simulink model "SCR_SiLS_R4_D101"  (R2023a)
settings: Solver=VariableStepAuto  StartTime=0.0  StopTime=T_sim_end  RelTol=1e-3
model workspace (MAT data in the model file):
  ConnVar.ipAddress = '192.168.0.153'
  ConnVar.user = 'M1'
  ConnVar.pwd = [145 145 158 146 151 156 158 157]
  ConnVar.targetHandle = 0
libraries: M1SWBlocks x6, simulink x6
settings Model: Creator=CHSE  LastModifiedBy=gione
settings DebuggingCC: UnconnectedInputMsg=warning  UnconnectedOutputMsg=warning  UnconnectedLineMsg=warning
settings ModelReferenceCC: EnableRefExpFcnMdlSchedulingChecks=on
settings RTWCC: DLArmComputeVersion=19.05

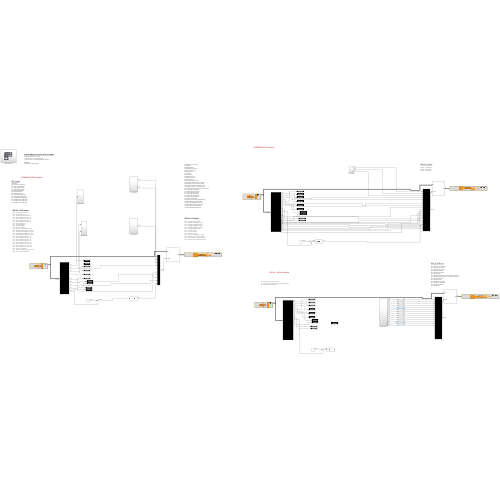
[thumbnail: Simulink's stored preview of the top-level diagram]
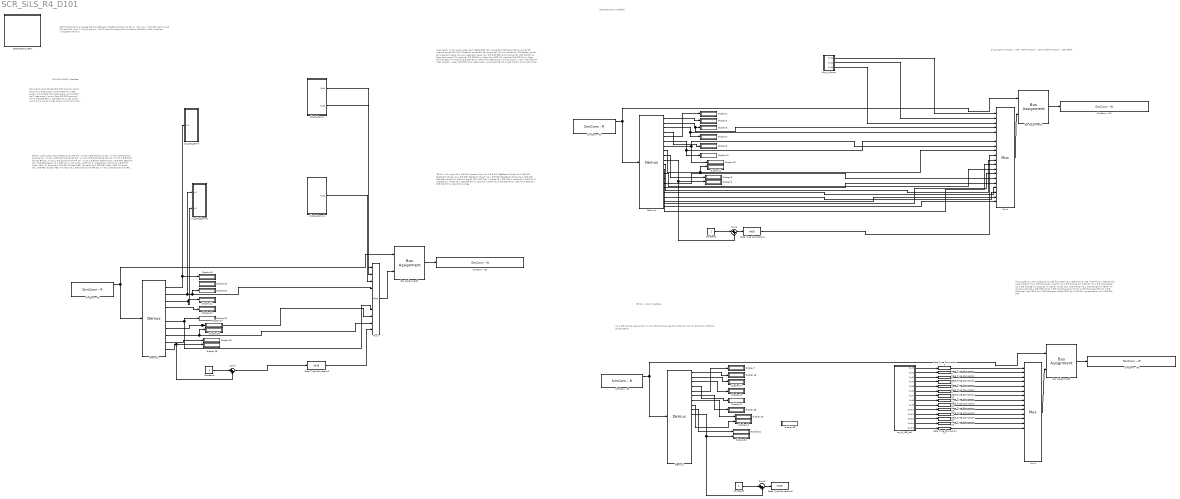
== system SCR_SiLS_R4_D101 ==
  note: No.1 G/E Dosing urea control VV
      |
      | No.1 G/E Dosing urea flow rate (l/h) (KR, NK class)
      |
      | No.1 G/E NOx concentration
  note: GE No. 1 DI intput
      |
      | No.1 G/E NOx sensor Alarm
      |
      | No.1 G/E RSV Feedback (Open)
      |
      | No.1 G/E RSV Feedback (Close)
      |
      | No.1 G/E RBV Feedback (Open)
      |
      | No.1 G/E RBV Feedback (Close)
      |
      | No.1 G/E SCR Remote mode
      |
      | No.1 G/E Run signal
      |
      | No.1 G/E Tier III mode
      |
      | No.1 G/E Tier II mode
      |
      | No.1 G/E Tier III preparation mode
      |
      | No.1 G/E SCR Em'cy stop from panel
      |
      | No.1 G/E SCR Emc'y stop from ECR
      |
      | No.1 G/E SCR Em'cy stop from bridge
  note: GE No. 1 DO output
      |
      | No.1 G/E Dosing urea Sol. VV
      |
      | No.1 G/E Dosing air Sol. VV
      |
      | No.1 G/E Dosing purging Sol. VV
      |
      | No.1 G/E Soot blower #1 Sol. VV
      |
      | No.1 G/E Soot blower #2 Sol. VV
      |
      | No.1 G/E Soot blower #3 Sol. VV
      |
      | No.1 G/E Soot blower #4 Sol. VV
      |
      | No.1 G/E RSV Setpoint
      |
      | No.1 G/E RBV Setpoint
      |
      | No.1 G/E SCR Ready
      |
      | No.1 G/E Tier III Active
      |
      | No.1 G/E Tier III preparation Active
      |
      | No.1 G/E RSV Open (ABS, NK class)
      |
      | No.1 G/E RSV Closed (ABS, NK class)
      |
      | No.1 G/E RBV Open (ABS, NK class)
      |
      | No.1 G/E RBV Closed (ABS, NK class)
      |
      | No.1 G/E Soot blower #5 Sol. VV
      |
      | No.1 G/E Soot blower #6 Sol. VV
      |
      | No.1 G/E Soot blower #7 Sol. VV
      |
      | No.1 G/E Soot blower #8 Sol. VV
      |
      | No.1 G/E Soot blower #9 Sol. VV
      |
      | No.1 G/E Soot blower #10 Sol. VV
      |
      | No.1 G/E Soot blower #11 Sol. VV
      |
      | No.1 G/E Soot blower #12 Sol. VV
      |
      | No.1 G/E Tier III Transfer
      |
      | No.1 SCR both bypass valve not open
      |
      | No.# G/E Common Shutdown
  note: DO output
      | Alarm Buzzer
      |
      | G/E SCR common alarm lamp
      |
      | No.1 Urea supply pump Start
      |
      | No.1 Urea supply pump Stop
      |
      | No.2 Urea supply pump Start
      |
      | No.2 Urea supply pump Stop
      |
      | G/E SCR common Alarm
      |
      | G/E SCR Em'cy Stopped
      |
      | No.1 Urea supply pump Running
      |
      | No.2 Urea supply pump Running
      |
      | No.1 G/E SCR Common Alarm lamp
      |
      | No.2 G/E SCR Common Alarm lamp
      |
      | No.3 G/E SCR Common Alarm lamp
      |
      | No.4 G/E SCR Common Alarm lamp
      |
      | ​
      |
      | ​
  note: Urea supply pump Auto mode
      |
      | Alarm Reset
      |
      | SCR Main power fail
      |
      | SCR Redundancy power fail
      |
      | Internal power fail(삭제됨)
      |
      | External power fail
      |
      | Fan power fail
      |
      | DC low insulation
      |
      | UPS battery power fail
      |
      | Urea tank Level Low-Low
      |
      | Urea tank Level Low
      |
      | G/E SCR ESD circuit power fail
      |
      | G/E SCR Em'cy Stop From panel (To module)
      |
      | G/E SCR Em'cy Stop From ECR (To module)
      |
      | G/E SCR Em'cy Stop From Bridge (To module)
      |
      | G/E SCR Em'cy Stop From Near Supply pump
      |
      | Supply, urea inlet filter dP High (Supply, urea inlet PDS)
      |
      | No.1 Urea supply pump Remote
      |
      | No.1 Urea supply pump Abnormal
      |
      | No.1 Urea supply pump Running
      |
      | No.2 Urea supply pump Remote
      |
      | No.2 Urea supply pump Abnormal
      |
      | No.2 Urea supply pump Running
      |
      | G/E Low Sulfur fuel supplied
      |
      | Urea tank drip tray Level High-High (ABS class)
      |
      | Urea tank TEMP High-High (ABS class)
      |
      | Urea tank Level High (ABS, BV, NK class)
      |
      | Urea tank drip tray Level High (ABS class)
      |
      | Urea tank TEMP Low (ABS, NK class)
      |
      | Urea tank TEMP High (ABS, NK class)
      |
      | ​
      |
      | ​
  note: COMMON DO/DI Interface
  note: SCR SiLS Model to evaluate the PLC software
      | modified at 2024.04.18. by Y.B. Kim
      |
      | -> Sils_DO_Comm: PLC DO and Sils input
      | -> Sils_DI_Comm : PLC DI and Sils output for simulation
      |
      | REMARK!!!
      | first, initialize workspace memory
  note: COMMON AO/AI Interface
  note: Sils_AI_Comm
      |
      | Supply, urea inlet PT
      |
      | Supply, urea outlet PT
      |
      | Supply, urea TEMP
  note: Sils_AI_GE no 1
      |
      | No.1 G/E Dosing urea flowmeter
      |
      | No.1 G/E Dosing urea inlet PT
      |
      | No.1 G/E Dosing urea outlet PT
      |
      | No.1 G/E Dosing air inlet PT
      |
      | No.1 G/E Dosing air outlet PT
      |
      | No.1 G/E Load signal
      |
      | No.1 G/E Charge Air pressure, Air cooler outlet (No.1 G/E PT212)
      |
      | No.1 G/E Charge Air TEMP, Air cooler outlet (No.1 G/E TE212)
      |
      | No.1 G/E Soot blower air PT
      |
      | No.1 G/E Chamber PDT
      |
      | No.1 G/E Chamber inlet TEMP
      |
      | No.1 G/E Chamber outlet TEMP
      |
      | No.1 G/E NOx concentration
      |
      | No.1 G/E RBV PDT
      |
      | ​
      |
      | ​
  note: GE No. 1 AO/AI Interface
  Bus Assignment1 : BusAssignment  AssignedSignals=data
  Bus Assignment2 : BusAssignment  AssignedSignals=data
  Bus Assignment3 : BusAssignment  AssignedSignals=data
  Constant1 : Constant
  Constant2 : Constant
  Constant3 : Constant
  Dashboard-system : Subsystem
  Data Type Conversion{1..17} (17 alike) : DataTypeConversion  OutDataTypeStr=int16  SaturateOnIntegerOverflow=off  RndMeth=Floor
  Demux1 : Demux  Outputs=20
  Demux2 : Demux  Outputs=10
  Demux4 : Demux  Outputs=20
  Display{1..5,7..32} (31 alike) : Display
      Display17 settings: Format=decimal (Stored Integer)
      Display20 settings: Format=decimal (Stored Integer)
      Display3 settings: Format=decimal (Stored Integer)
  Mux1 : Mux  Inputs=20
  Mux2 : Mux  Inputs=10
  Mux4 : Mux  Inputs=20
  SimConn - R1 : M1SWBlocks/SimConn Blocks/SimConn - R  connVarName=ConnVar  InswModuleName='NONOXR4'  swModuleName=NONOXR4  InvarName='.Sils_AO_Comm'  varName=.Sils_AO_Comm  varDataType=Bus: IOSim_AIO_typ  enRetOutput=on  enGetTrigger=off  getTrigger=rising  valDurLostConn=Zero  internalVal=0  DataDim=1  enSampTimMon=on  sampleTime=Ts_com
      settings: SourceProductName=Bachmann M1 Software
  SimConn - R2 : M1SWBlocks/SimConn Blocks/SimConn - R  connVarName=ConnVar  InswModuleName='NONOXR4'  swModuleName=NONOXR4  InvarName='.Sils_DO_Comm'  varName=.Sils_DO_Comm  varDataType=Bus: IOSim_typ  enRetOutput=on  enGetTrigger=off  getTrigger=rising  valDurLostConn=Zero  internalVal=0  DataDim=1  enSampTimMon=on  sampleTime=Ts_com
      settings: SourceProductName=Bachmann M1 Software
  SimConn - R3 : M1SWBlocks/SimConn Blocks/SimConn - R  connVarName=ConnVar  InswModuleName='NONOXR4'  swModuleName=NONOXR4  InvarName='.Sils_AO_GE1'  varName=.Sils_AO_GE1  varDataType=Bus: IOSim_AIO_typ  enRetOutput=on  enGetTrigger=off  getTrigger=rising  valDurLostConn=Zero  internalVal=0  DataDim=1  enSampTimMon=on  sampleTime=Ts_com
      settings: SourceProductName=Bachmann M1 Software
  SimConn - W1 : M1SWBlocks/SimConn Blocks/SimConn - W  connVarName=ConnVar  InswModuleName='NONOXR4'  swModuleName=NONOXR4  InvarName='.Sils_AI_Comm'  varName=.Sils_AI_Comm  varDataType=Bus: IOSim_AIO_typ  enRetOutput=off  enGetTrigger=off  getTrigger=rising  enSampTimMon=off
      settings: SourceProductName=Bachmann M1 Software
  SimConn - W2 : M1SWBlocks/SimConn Blocks/SimConn - W  connVarName=ConnVar  InswModuleName='NONOXR4'  swModuleName=NONOXR4  InvarName='.Sils_DI_Comm'  varName=.Sils_DI_Comm  varDataType=Bus: IOSim_typ  enRetOutput=off  enGetTrigger=off  getTrigger=rising  enSampTimMon=off
      settings: SourceProductName=Bachmann M1 Software
  SimConn - W3 : M1SWBlocks/SimConn Blocks/SimConn - W  connVarName=ConnVar  InswModuleName='NONOXR4'  swModuleName=NONOXR4  InvarName='.Sils_AI_GE1'  varName=.Sils_AI_GE1  varDataType=Bus: IOSim_AIO_typ  enRetOutput=off  enGetTrigger=off  getTrigger=rising  enSampTimMon=off
      settings: SourceProductName=Bachmann M1 Software
  Sum1 : Sum  Inputs=|++
  Sum2 : Sum  Inputs=|++
  Sum3 : Sum  Inputs=|++
  sils_AI_Comm : Subsystem
  sils_AI_GE_No1 : Subsystem
  sils_DI_Comm : Subsystem
  sils_DI_Comm1 : Subsystem
  sils_DO_Comm : Subsystem
  sils_DO_Comm1 : Subsystem
  wires:
  Demux2/3 -> sils_DO_Comm1/2(In2), Display21/1
  Constant1/1 -> Sum1/1
  Demux2/4 -> Display22/1
  Sum1/1 -> Data Type Conversion2/1
  Demux2/2 -> Mux2/4, Display20/1, sils_DO_Comm1/1(In1)
  SimConn - R2/1 -> Bus Assignment2/1, Demux2/1
  Demux2/9 -> Display25/1
  Demux2/10 -> Sum1/2, Display26/1
  Demux2/8 -> Mux2/9, Display28/1
  Demux2/7 -> Mux2/8, Display27/1
  Demux2/6 -> Mux2/7, Display29/1
  Mux2/1 -> Bus Assignment2/2
  Bus Assignment2/1 -> SimConn - W2/1
  Data Type Conversion2/1 -> Mux2/10
  Demux4/6 -> Display12/1, Mux4/7
  Bus Assignment1/1 -> SimConn - W1/1
  Demux4/9 -> Display8/1
  Demux4/7 -> Display10/1, Mux4/8
  Mux4/1 -> Bus Assignment1/2
  Demux4/10 -> Sum2/2, Display9/1
  Demux4/1 -> Display2/1
  Data Type Conversion1/1 -> Mux4/10
  Demux4/8 -> Mux4/9, Display11/1
  Demux4/5 -> Display1/1
  SimConn - R1/1 -> Bus Assignment1/1, Demux4/1
  Demux4/4 -> Display5/1
  Demux4/2 -> Mux4/4, Display3/1
  Sum2/1 -> Data Type Conversion1/1
  Constant2/1 -> Sum2/1
  Demux4/3 -> Display4/1, Mux4/5
  Demux4/11 -> Mux4/11
  Demux4/12 -> Mux4/12
  Demux4/13 -> Mux4/13
  Demux4/14 -> Mux4/14
  Demux4/15 -> Mux4/15
  Demux4/16 -> Mux4/16
  Demux4/17 -> Mux4/17
  Demux4/18 -> Mux4/18
  Demux4/19 -> Mux4/19
  Demux4/20 -> Mux4/20
  Demux2/1 -> sils_DO_Comm/1(In1), Display18/1
  sils_DI_Comm/1(Out2) -> Mux2/1
  sils_DI_Comm/2(Out3) -> Mux2/2
  sils_AI_Comm/1(Out1) -> Mux4/1
  sils_AI_Comm/2(Out2) -> Mux4/2
  sils_AI_Comm/3(Out3) -> Mux4/3
  sils_DI_Comm1/1(Out2) -> Mux2/3
  Constant3/1 -> Sum3/1
  Demux1/1 -> Display16/1
  Demux1/4 -> Display24/1
  Demux1/5 -> Display7/1
  Demux1/2 -> Display17/1
  Demux1/9 -> Display31/1
  Mux1/1 -> Bus Assignment3/2
  Bus Assignment3/1 -> SimConn - W3/1
  Demux1/6 -> Display15/1
  Sum3/1 -> Data Type Conversion3/1
  Demux1/8 -> Display14/1
  Demux1/7 -> Display13/1
  SimConn - R3/1 -> Bus Assignment3/1, Demux1/1
  Demux1/3 -> Display23/1
  sils_AI_GE_No1/3(Out3) -> Data Type Conversion6/1
  sils_AI_GE_No1/1(Out1) -> Data Type Conversion4/1
  sils_AI_GE_No1/2(Out2) -> Data Type Conversion5/1
  Demux1/10 -> Sum3/2, Display32/1
  sils_AI_GE_No1/4(Out4) -> Data Type Conversion7/1
  sils_AI_GE_No1/5(Out5) -> Data Type Conversion8/1
  sils_AI_GE_No1/6(Out6) -> Data Type Conversion9/1
  sils_AI_GE_No1/7(Out7) -> Data Type Conversion10/1
  sils_AI_GE_No1/8(Out8) -> Data Type Conversion11/1
  sils_AI_GE_No1/9(Out9) -> Data Type Conversion12/1
  sils_AI_GE_No1/10(Out10) -> Data Type Conversion13/1
  sils_AI_GE_No1/11(Out11) -> Data Type Conversion14/1
  sils_AI_GE_No1/12(Out12) -> Data Type Conversion15/1
  sils_AI_GE_No1/14(Out13) -> Data Type Conversion17/1
  sils_AI_GE_No1/13(Out14) -> Data Type Conversion16/1
  Data Type Conversion4/1 -> Mux1/1
  Data Type Conversion5/1 -> Mux1/2
  Data Type Conversion6/1 -> Mux1/3
  Data Type Conversion9/1 -> Mux1/6
  Data Type Conversion8/1 -> Mux1/5
  Data Type Conversion7/1 -> Mux1/4
  Data Type Conversion10/1 -> Mux1/7
  Data Type Conversion11/1 -> Mux1/8
  Data Type Conversion12/1 -> Mux1/9
  Data Type Conversion13/1 -> Mux1/10
  Data Type Conversion14/1 -> Mux1/11
  Data Type Conversion15/1 -> Mux1/12
  Data Type Conversion16/1 -> Mux1/13
  Data Type Conversion17/1 -> Mux1/14

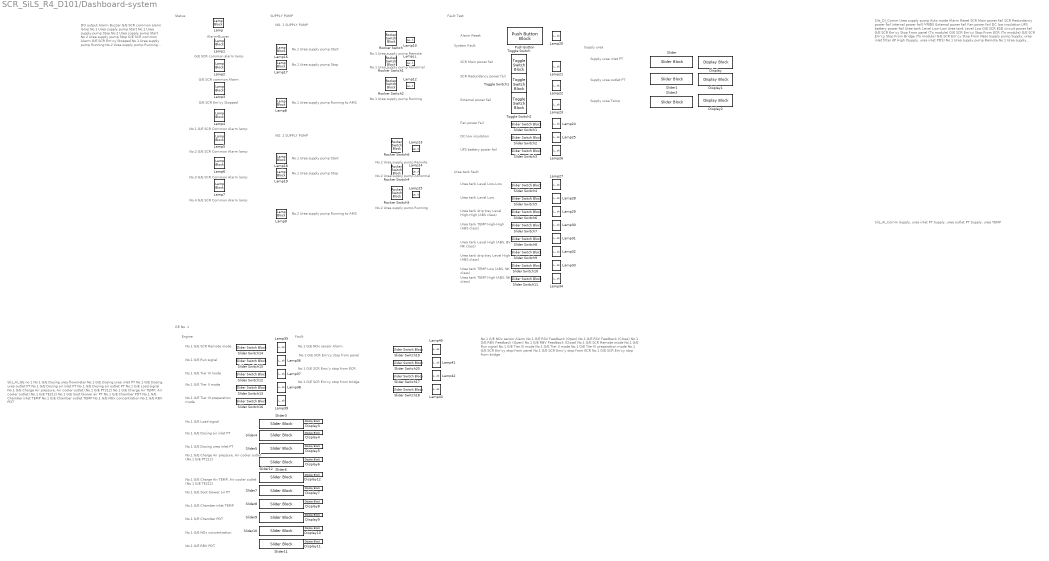
== system SCR_SiLS_R4_D101/Dashboard-system ==
  note: Fault
  note: Engine
  note: GE No. 1
  note: Supply urea
  note: Urea tank fault
  note: System Fault
  note: NO. 1 SUPPLY PUMP
  note: SUPPLY PUMP
  note: Alarm Buzzer
  note: G/E SCR common alarm lamp
  note: DO output
      | Alarm Buzzer
      |
      | G/E SCR common alarm lamp
      |
      | No.1 Urea supply pump Start
      |
      | No.1 Urea supply pump Stop
      |
      | No.2 Urea supply pump Start
      |
      | No.2 Urea supply pump Stop
      |
      | G/E SCR common Alarm
      |
      | G/E SCR Em'cy Stopped
      |
      | No.1 Urea supply pump Running
      |
      | No.2 Urea supply pump Running
      |
      | No.1 G/E SCR Common Alarm lamp
      |
      | No.2 G/E SCR Common Alarm lamp
      |
      | No.3 G/E SCR Common Alarm lamp
      |
      | No.4 G/E SCR Common Alarm lamp
      |
      | ​
      |
      | ​
  note: G/E SCR Em'cy Stopped
  note: G/E SCR common Alarm
  note: No.1 G/E SCR Common Alarm lamp
  note: No.2 G/E SCR Common Alarm lamp
  note: No.3 G/E SCR Common Alarm lamp
  note: No.4 G/E SCR Common Alarm lamp
  note: Status
  note: No.1 Urea supply pump Running to AMS
  note: NO. 2 SUPPLY PUMP
  note: No.2 Urea supply pump Running to AMS
  note: No.1 Urea supply pump Remote
  note: No.1 Urea supply pump Abnormal
  note: No.1 Urea supply pump Running
  note: Sils_DI_Comm
      |
      | Urea supply pump Auto mode
      |
      | Alarm Reset
      |
      | SCR Main power fail
      |
      | SCR Redundancy power fail
      |
      | Internal power fail(삭제됨)
      |
      | External power fail
      |
      | Fan power fail
      |
      | DC low insulation
      |
      | UPS battery power fail
      |
      | Urea tank Level Low-Low
      |
      | Urea tank Level Low
      |
      | G/E SCR ESD circuit power fail
      |
      | G/E SCR Em'cy Stop From panel (To module)
      |
      | G/E SCR Em'cy Stop From ECR (To module)
      |
      | G/E SCR Em'cy Stop From Bridge (To module)
      |
      | G/E SCR Em'cy Stop From Near Supply pump
      |
      | Supply, urea inlet filter dP High (Supply, urea inlet PDS)
      |
      | No.1 Urea supply pump Remote
      |
      | No.1 Urea supply pump Abnormal
      |
      | No.1 Urea supply pump Running
      |
      | No.2 Urea supply pump Remote
      |
      | No.2 Urea supply pump Abnormal
      |
      | No.2 Urea supply pump Running
      |
      | G/E Low Sulfur fuel supplied
      |
      | Urea tank drip tray Level High-High (ABS class)
      |
      | Urea tank TEMP High-High (ABS class)
      |
      | Urea tank Level High (ABS, BV, NK class)
      |
      | Urea tank drip tray Level High (ABS class)
      |
      | Urea tank TEMP Low (ABS, NK class)
      |
      | Urea tank TEMP High (ABS, NK class)
      |
      | ​
      |
      | ​
  note: No.2 Urea supply pump Running
  note: No.2 Urea supply pump Abnormal
  note: No.2 Urea supply pump Remote
  note: No.1 Urea supply pump Start
  note: No.1 Urea supply pump Stop
  note: No.1 Urea supply pump Stop
  note: No.1 Urea supply pump Start
  note: Fault Test
  note: Alarm Reset
  note: SCR Main power fail
  note: SCR Redundancy power fail
  note: External power fail
  note: Fan power fail
  note: DC low insulation
  note: UPS battery power fail
  note: Urea tank Level Low-Low
  note: Urea tank Level Low
  note: Urea tank drip tray Level High-High (ABS class)
  note: Urea tank TEMP High-High (ABS class)
  note: Urea tank Level High (ABS, BV, NK class)
  note: Urea tank drip tray Level High (ABS class)
  note: Urea tank TEMP Low (ABS, NK class)
  note: Urea tank TEMP High (ABS, NK class)
  note: Supply urea inlet PT
  note: Sils_AI_Comm
      |
      | Supply, urea inlet PT
      |
      | Supply, urea outlet PT
      |
      | Supply, urea TEMP
  note: Supply urea outlet PT
  note: Supply urea Temp
  note: No.1 G/E NOx sensor Alarm
      |
      | No.1 G/E RSV Feedback (Open)
      |
      | No.1 G/E RSV Feedback (Close)
      |
      | No.1 G/E RBV Feedback (Open)
      |
      | No.1 G/E RBV Feedback (Close)
      |
      | No.1 G/E SCR Remote mode
      |
      | No.1 G/E Run signal
      |
      | No.1 G/E Tier III mode
      |
      | No.1 G/E Tier II mode
      |
      | No.1 G/E Tier III preparation mode
      |
      | No.1 G/E SCR Em'cy stop from panel
      |
      | No.1 G/E SCR Emc'y stop from ECR
      |
      | No.1 G/E SCR Em'cy stop from bridge
  note: No.1 G/E Tier II mode
  note: No.1 G/E Tier III mode
  note: No.1 G/E Run signal
  note: No.1 G/E SCR Remote mode
  note: No.1 G/E Tier III preparation mode
  note: No.1 G/E SCR Emc'y stop from ECR
  note: No.1 G/E SCR Em'cy stop from bridge
  note: No.1 G/E NOx sensor Alarm
  note: No.1 G/E SCR Em'cy stop from panel
  note: No.1 G/E Load signal
  note: Sils_AI_GE no 1
      |
      | No.1 G/E Dosing urea flowmeter
      |
      | No.1 G/E Dosing urea inlet PT
      |
      | No.1 G/E Dosing urea outlet PT
      |
      | No.1 G/E Dosing air inlet PT
      |
      | No.1 G/E Dosing air outlet PT
      |
      | No.1 G/E Load signal
      |
      | No.1 G/E Charge Air pressure, Air cooler outlet (No.1 G/E PT212)
      |
      | No.1 G/E Charge Air TEMP, Air cooler outlet (No.1 G/E TE212)
      |
      | No.1 G/E Soot blower air PT
      |
      | No.1 G/E Chamber PDT
      |
      | No.1 G/E Chamber inlet TEMP
      |
      | No.1 G/E Chamber outlet TEMP
      |
      | No.1 G/E NOx concentration
      |
      | No.1 G/E RBV PDT
      |
      | ​
      |
      | ​
  note: No.1 G/E Dosing air inlet PT
  note: No.1 G/E Dosing urea inlet PT
  note: No.1 G/E Charge Air pressure, Air cooler outlet (No.1 G/E PT212)
  note: No.1 G/E Soot blower air PT
  note: No.1 G/E Chamber inlet TEMP
  note: No.1 G/E Chamber PDT
  note: No.1 G/E NOx concentration
  note: No.1 G/E RBV PDT
  note: No.1 G/E Charge Air TEMP, Air cooler outlet (No.1 G/E TE212)
  Display{,1..12} (13 alike) : DisplayBlock  LabelPosition=Hide  Transparency=1
  Lamp{,1..43} (44 alike) : LampBlock  LabelPosition=Hide
  Push Button : PushButtonBlock  ButtonText=Alarm Reset  OffValue=0.000000
  Rocker Switch{,1..2,4..6} (6 alike) : RockerSwitchBlock  LabelPosition=Hide
      settings: Values={{'Off', 'On'}, [0 1]}
  Slider : SliderBlock  LabelPosition=Hide  ScaleMax=16
  Slider Switch{1..20} (20 alike) : SliderSwitchBlock  LabelPosition=Hide
      settings: Values={{'Off', 'On'}, [0 1]}
  Slider1 : SliderBlock  LabelPosition=Hide  ScaleMax=16
  Slider10 : SliderBlock  LabelPosition=Hide  ScaleMax=120
  Slider11 : SliderBlock  LabelPosition=Hide
  Slider12 : SliderBlock  LabelPosition=Hide  ScaleMax=200
  Slider2 : SliderBlock  LabelPosition=Hide
  Slider3 : SliderBlock  LabelPosition=Hide  ScaleMax=120
  Slider4 : SliderBlock  LabelPosition=Hide  ScaleMax=15
  Slider5 : SliderBlock  LabelPosition=Hide  ScaleMax=15
  Slider6 : SliderBlock  LabelPosition=Hide  ScaleMax=10
  Slider7 : SliderBlock  LabelPosition=Hide  ScaleMax=120
  Slider8 : SliderBlock  LabelPosition=Hide  ScaleMax=600
  Slider9 : SliderBlock  LabelPosition=Hide
  Toggle Switch : ToggleSwitchBlock  LabelPosition=Hide
      settings: Values={{'Off', 'On'}, [0 1]}
  Toggle Switch1 : ToggleSwitchBlock  LabelPosition=Hide
      settings: Values={{'Off', 'On'}, [0 1]}
  Toggle Switch2 : ToggleSwitchBlock  LabelPosition=Hide
      settings: Values={{'Off', 'On'}, [0 1]}

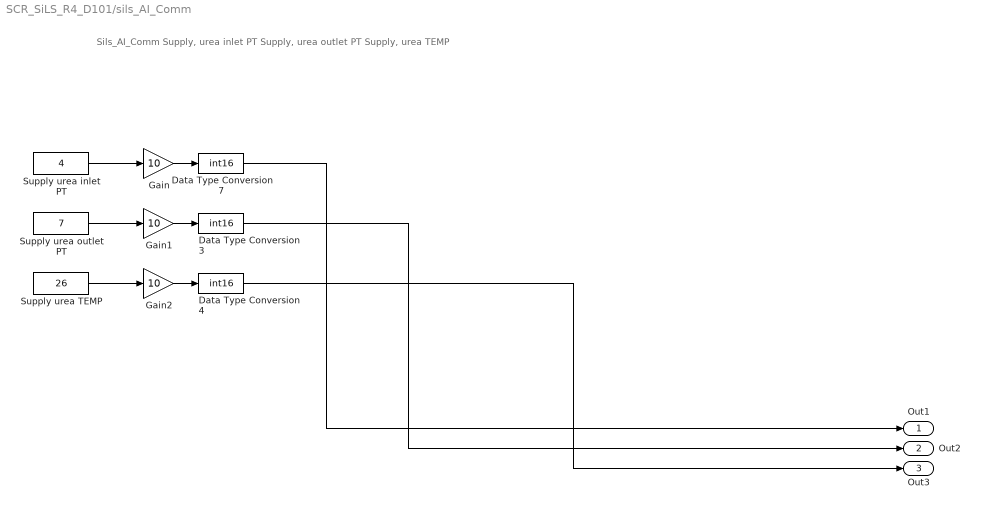
== system SCR_SiLS_R4_D101/sils_AI_Comm ==
  note: Sils_AI_Comm
      |
      | Supply, urea inlet PT
      |
      | Supply, urea outlet PT
      |
      | Supply, urea TEMP
  Data Type Conversion3 : DataTypeConversion  OutDataTypeStr=int16  SaturateOnIntegerOverflow=off  RndMeth=Floor
  Data Type Conversion4 : DataTypeConversion  OutDataTypeStr=int16  SaturateOnIntegerOverflow=off  RndMeth=Floor
  Data Type Conversion7 : DataTypeConversion  OutDataTypeStr=int16  SaturateOnIntegerOverflow=off  RndMeth=Floor
  Gain : Gain  Gain=10
  Gain1 : Gain  Gain=10
  Gain2 : Gain  Gain=10
  Supply urea TEMP : Constant  Value=26
  Supply urea inlet PT : Constant  Value=4
  Supply urea outlet PT : Constant  Value=7
  Out1 : Outport
  Out2 : Outport  Port=2
  Out3 : Outport  Port=3
  wires:
  Supply urea inlet PT/1 -> Gain/1
  Supply urea outlet PT/1 -> Gain1/1
  Gain1/1 -> Data Type Conversion3/1
  Data Type Conversion3/1 -> Out2/1
  Supply urea TEMP/1 -> Gain2/1
  Gain2/1 -> Data Type Conversion4/1
  Gain/1 -> Data Type Conversion7/1
  Data Type Conversion7/1 -> Out1/1
  Data Type Conversion4/1 -> Out3/1

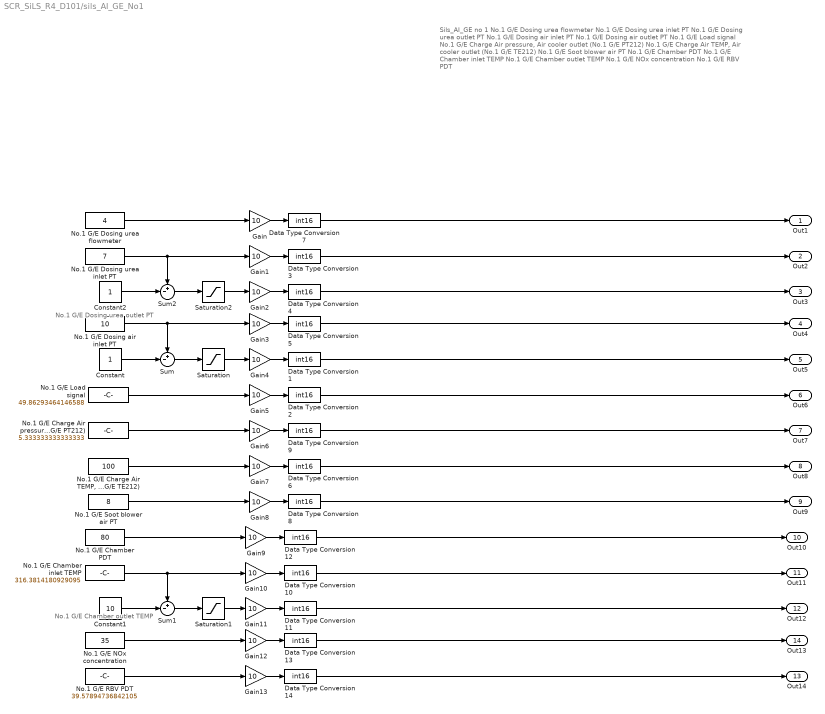
== system SCR_SiLS_R4_D101/sils_AI_GE_No1 ==
  note: No.1 G/E Dosing urea outlet PT
  note: No.1 G/E Chamber outlet TEMP
  note: Sils_AI_GE no 1
      |
      | No.1 G/E Dosing urea flowmeter
      |
      | No.1 G/E Dosing urea inlet PT
      |
      | No.1 G/E Dosing urea outlet PT
      |
      | No.1 G/E Dosing air inlet PT
      |
      | No.1 G/E Dosing air outlet PT
      |
      | No.1 G/E Load signal
      |
      | No.1 G/E Charge Air pressure, Air cooler outlet (No.1 G/E PT212)
      |
      | No.1 G/E Charge Air TEMP, Air cooler outlet (No.1 G/E TE212)
      |
      | No.1 G/E Soot blower air PT
      |
      | No.1 G/E Chamber PDT
      |
      | No.1 G/E Chamber inlet TEMP
      |
      | No.1 G/E Chamber outlet TEMP
      |
      | No.1 G/E NOx concentration
      |
      | No.1 G/E RBV PDT
      |
      | ​
      |
      | ​
  Constant : Constant
  Constant1 : Constant  Value=10
  Constant2 : Constant
  Data Type Conversion{1..14} (14 alike) : DataTypeConversion  OutDataTypeStr=int16  SaturateOnIntegerOverflow=off  RndMeth=Floor
  Gain{,1..13} (14 alike) : Gain  Gain=10
  No.1 G/E Chamber PDT : Constant  Value=80
  No.1 G/E Chamber inlet TEMP : Constant  Value=316.3814180929095
  "No.1 G/E Charge Air TEMP, Air cooler outlet (No.1 G/E TE212)" : Constant  Value=100
  "No.1 G/E Charge Air pressure, Air cooler outlet (No.1 G/E PT212)" : Constant  Value=5.333333333333333
  No.1 G/E Dosing air inlet PT : Constant  Value=10
  No.1 G/E Dosing urea flowmeter : Constant  Value=4
  No.1 G/E Dosing urea inlet PT : Constant  Value=7
  No.1 G/E Load signal : Constant  Value=49.86293464146588
  No.1 G/E NOx concentration : Constant  Value=35
  No.1 G/E RBV PDT : Constant  Value=39.57894736842105
  No.1 G/E Soot blower air PT : Constant  Value=8
  Saturation : Saturate  UpperLimit=10.0  LowerLimit=0.0
  Saturation1 : Saturate  UpperLimit=500.0  LowerLimit=0.0
  Saturation2 : Saturate  UpperLimit=10.0  LowerLimit=0.0
  Sum : Sum  Inputs=+-|
  Sum1 : Sum  Inputs=+-|
  Sum2 : Sum  Inputs=+-|
  Out1 : Outport
  Out2 : Outport  Port=2
  Out3 : Outport  Port=3
  Out4 : Outport  Port=4
  Out5 : Outport  Port=5
  Out6 : Outport  Port=6
  Out7 : Outport  Port=7
  Out8 : Outport  Port=8
  Out9 : Outport  Port=9
  Out10 : Outport  Port=10
  Out11 : Outport  Port=11
  Out12 : Outport  Port=12
  Out14 : Outport  Port=13
  Out13 : Outport  Port=14
  wires:
  No.1 G/E Dosing urea flowmeter/1 -> Gain/1
  Gain1/1 -> Data Type Conversion3/1
  Data Type Conversion3/1 -> Out2/1
  Gain2/1 -> Data Type Conversion4/1
  Gain/1 -> Data Type Conversion7/1
  Data Type Conversion7/1 -> Out1/1
  Data Type Conversion4/1 -> Out3/1
  No.1 G/E Dosing air inlet PT/1 -> Gain3/1, Sum/1
  Gain4/1 -> Data Type Conversion1/1
  Sum/1 -> Saturation/1
  No.1 G/E Load signal/1 -> Gain5/1
  Data Type Conversion5/1 -> Out4/1
  Data Type Conversion1/1 -> Out5/1
  Data Type Conversion2/1 -> Out6/1
  Gain3/1 -> Data Type Conversion5/1
  Gain5/1 -> Data Type Conversion2/1
  "No.1 G/E Charge Air pressure, Air cooler outlet (No.1 G/E PT212)"/1 -> Gain6/1
  Gain7/1 -> Data Type Conversion6/1
  "No.1 G/E Charge Air TEMP, Air cooler outlet (No.1 G/E TE212)"/1 -> Gain7/1
  No.1 G/E Soot blower air PT/1 -> Gain8/1
  Data Type Conversion9/1 -> Out7/1
  Data Type Conversion6/1 -> Out8/1
  Data Type Conversion8/1 -> Out9/1
  Gain6/1 -> Data Type Conversion9/1
  Gain8/1 -> Data Type Conversion8/1
  No.1 G/E Chamber PDT/1 -> Gain9/1
  Gain10/1 -> Data Type Conversion10/1
  No.1 G/E Chamber inlet TEMP/1 -> Sum1/1, Gain10/1
  Data Type Conversion12/1 -> Out10/1
  Data Type Conversion10/1 -> Out11/1
  Data Type Conversion11/1 -> Out12/1
  Gain9/1 -> Data Type Conversion12/1
  Gain11/1 -> Data Type Conversion11/1
  No.1 G/E RBV PDT/1 -> Gain13/1
  Data Type Conversion14/1 -> Out14/1
  Data Type Conversion13/1 -> Out13/1
  Gain12/1 -> Data Type Conversion13/1
  Gain13/1 -> Data Type Conversion14/1
  No.1 G/E NOx concentration/1 -> Gain12/1
  Constant/1 -> Sum/2
  Saturation/1 -> Gain4/1
  Sum1/1 -> Saturation1/1
  Constant1/1 -> Sum1/2
  Saturation1/1 -> Gain11/1
  No.1 G/E Dosing urea inlet PT/1 -> Gain1/1, Sum2/1
  Sum2/1 -> Saturation2/1
  Constant2/1 -> Sum2/2
  Saturation2/1 -> Gain2/1

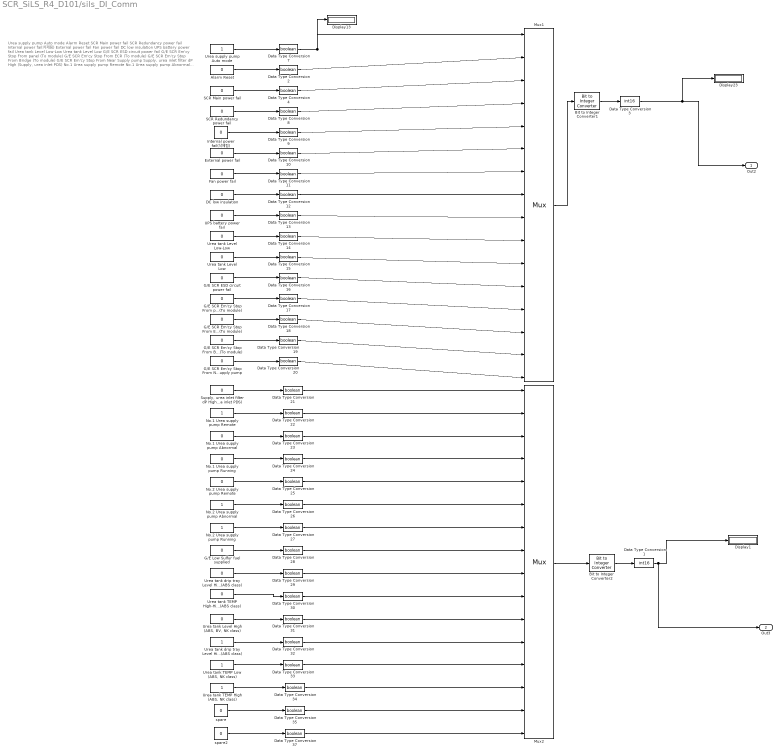
== system SCR_SiLS_R4_D101/sils_DI_Comm ==
  note: Urea supply pump Auto mode
      |
      | Alarm Reset
      |
      | SCR Main power fail
      |
      | SCR Redundancy power fail
      |
      | Internal power fail(삭제됨)
      |
      | External power fail
      |
      | Fan power fail
      |
      | DC low insulation
      |
      | UPS battery power fail
      |
      | Urea tank Level Low-Low
      |
      | Urea tank Level Low
      |
      | G/E SCR ESD circuit power fail
      |
      | G/E SCR Em'cy Stop From panel (To module)
      |
      | G/E SCR Em'cy Stop From ECR (To module)
      |
      | G/E SCR Em'cy Stop From Bridge (To module)
      |
      | G/E SCR Em'cy Stop From Near Supply pump
      |
      | Supply, urea inlet filter dP High (Supply, urea inlet PDS)
      |
      | No.1 Urea supply pump Remote
      |
      | No.1 Urea supply pump Abnormal
      |
      | No.1 Urea supply pump Running
      |
      | No.2 Urea supply pump Remote
      |
      | No.2 Urea supply pump Abnormal
      |
      | No.2 Urea supply pump Running
      |
      | G/E Low Sulfur fuel supplied
      |
      | Urea tank drip tray Level High-High (ABS class)
      |
      | Urea tank TEMP High-High (ABS class)
      |
      | Urea tank Level High (ABS, BV, NK class)
      |
      | Urea tank drip tray Level High (ABS class)
      |
      | Urea tank TEMP Low (ABS, NK class)
      |
      | Urea tank TEMP High (ABS, NK class)
      |
      | ​
      |
      | ​
  Alarm Reset : Constant  Value=0
  Bit to Integer Converter1 : simulink/Logic and Bit Operations/Bit to Integer Converter  nbits=16  bitOrder=LSB first  signedOutputValues=Unsigned  outDtype=Inherit via internal rule  outDtypeSigned=Inherit via internal rule
  Bit to Integer Converter2 : simulink/Logic and Bit Operations/Bit to Integer Converter  nbits=16  bitOrder=LSB first  signedOutputValues=Unsigned  outDtype=Inherit via internal rule  outDtypeSigned=Inherit via internal rule
  DC low insulation : Constant  Value=0
  Data Type Conversion1 : DataTypeConversion  OutDataTypeStr=int16  SaturateOnIntegerOverflow=off  RndMeth=Floor
  Data Type Conversion{2,4,7..35,37} (32 alike) : DataTypeConversion  OutDataTypeStr=boolean  SaturateOnIntegerOverflow=off  RndMeth=Floor
  Data Type Conversion3 : DataTypeConversion  OutDataTypeStr=int16  SaturateOnIntegerOverflow=off  RndMeth=Floor
  Display1 : Display
  Display13 : Display
  Display23 : Display
  External power fail : Constant  Value=0
  Fan power fail : Constant  Value=0
  G/E Low Sulfur fuel supplied : Constant  Value=0
  G/E SCR ESD circuit power fail : Constant  Value=0
  G/E SCR Em'cy Stop From Bridge (To module) : Constant  Value=0
  G/E SCR Em'cy Stop From ECR (To module) : Constant  Value=0
  G/E SCR Em'cy Stop From Near Supply pump : Constant  Value=0
  G/E SCR Em'cy Stop From panel (To module) : Constant  Value=0
  Internal power fail(삭제됨) : Constant  Value=0
  Mux1 : Mux  Inputs=16
  Mux2 : Mux  Inputs=16
  No.1 Urea supply pump Abnormal : Constant  Value=0
  No.1 Urea supply pump Remote : Constant
  No.1 Urea supply pump Running : Constant  Value=0
  No.2 Urea supply pump Abnormal : Constant
  No.2 Urea supply pump Remote : Constant  Value=0
  No.2 Urea supply pump Running : Constant
  SCR Main power fail : Constant  Value=0
  SCR Redundancy power fail : Constant  Value=0
  "Supply, urea inlet filter dP High (Supply, urea inlet PDS)" : Constant  Value=0
  UPS battery power fail : Constant  Value=0
  Urea supply pump Auto mode : Constant
  "Urea tank Level High (ABS, BV, NK class)" : Constant  Value=0
  Urea tank Level Low : Constant  Value=0
  Urea tank Level Low-Low : Constant  Value=0
  "Urea tank TEMP High (ABS, NK class)" : Constant
  Urea tank TEMP High-High (ABS class) : Constant  Value=0
  "Urea tank TEMP Low (ABS, NK class)" : Constant
  Urea tank drip tray Level High (ABS class) : Constant
  Urea tank drip tray Level High-High (ABS class) : Constant  Value=0
  spare : Constant  Value=0
  spare2 : Constant  Value=0
  Out2 : Outport
  Out3 : Outport  Port=2
  wires:
  Urea supply pump Auto mode/1 -> Data Type Conversion7/1
  Data Type Conversion7/1 -> Display13/1, Mux1/1
  Data Type Conversion3/1 -> Out2/1, Display23/1
  Bit to Integer Converter1/1 -> Data Type Conversion3/1
  Mux1/1 -> Bit to Integer Converter1/1
  Alarm Reset/1 -> Data Type Conversion2/1
  SCR Main power fail/1 -> Data Type Conversion4/1
  SCR Redundancy power fail/1 -> Data Type Conversion8/1
  Internal power fail(삭제됨)/1 -> Data Type Conversion9/1
  External power fail/1 -> Data Type Conversion10/1
  Fan power fail/1 -> Data Type Conversion11/1
  DC low insulation/1 -> Data Type Conversion12/1
  UPS battery power fail/1 -> Data Type Conversion13/1
  Urea tank Level Low-Low/1 -> Data Type Conversion14/1
  Urea tank Level Low/1 -> Data Type Conversion15/1
  G/E SCR ESD circuit power fail/1 -> Data Type Conversion16/1
  G/E SCR Em'cy Stop From panel (To module)/1 -> Data Type Conversion17/1
  G/E SCR Em'cy Stop From ECR (To module)/1 -> Data Type Conversion18/1
  G/E SCR Em'cy Stop From Bridge (To module)/1 -> Data Type Conversion19/1
  G/E SCR Em'cy Stop From Near Supply pump/1 -> Data Type Conversion20/1
  "Supply, urea inlet filter dP High (Supply, urea inlet PDS)"/1 -> Data Type Conversion21/1
  No.1 Urea supply pump Remote/1 -> Data Type Conversion22/1
  No.1 Urea supply pump Abnormal/1 -> Data Type Conversion23/1
  No.1 Urea supply pump Running/1 -> Data Type Conversion24/1
  No.2 Urea supply pump Remote/1 -> Data Type Conversion25/1
  No.2 Urea supply pump Abnormal/1 -> Data Type Conversion26/1
  No.2 Urea supply pump Running/1 -> Data Type Conversion27/1
  G/E Low Sulfur fuel supplied/1 -> Data Type Conversion28/1
  Urea tank drip tray Level High-High (ABS class)/1 -> Data Type Conversion29/1
  Urea tank TEMP High-High (ABS class)/1 -> Data Type Conversion30/1
  "Urea tank Level High (ABS, BV, NK class)"/1 -> Data Type Conversion31/1
  Urea tank drip tray Level High (ABS class)/1 -> Data Type Conversion32/1
  "Urea tank TEMP Low (ABS, NK class)"/1 -> Data Type Conversion33/1
  "Urea tank TEMP High (ABS, NK class)"/1 -> Data Type Conversion34/1
  spare/1 -> Data Type Conversion35/1
  spare2/1 -> Data Type Conversion37/1
  Data Type Conversion1/1 -> Out3/1, Display1/1
  Bit to Integer Converter2/1 -> Data Type Conversion1/1
  Mux2/1 -> Bit to Integer Converter2/1
  Data Type Conversion2/1 -> Mux1/2
  Data Type Conversion4/1 -> Mux1/3
  Data Type Conversion8/1 -> Mux1/4
  Data Type Conversion9/1 -> Mux1/5
  Data Type Conversion10/1 -> Mux1/6
  Data Type Conversion11/1 -> Mux1/7
  Data Type Conversion12/1 -> Mux1/8
  Data Type Conversion13/1 -> Mux1/9
  Data Type Conversion14/1 -> Mux1/10
  Data Type Conversion15/1 -> Mux1/11
  Data Type Conversion16/1 -> Mux1/12
  Data Type Conversion17/1 -> Mux1/13
  Data Type Conversion18/1 -> Mux1/14
  Data Type Conversion19/1 -> Mux1/15
  Data Type Conversion20/1 -> Mux1/16
  Data Type Conversion21/1 -> Mux2/1
  Data Type Conversion25/1 -> Mux2/5
  Data Type Conversion22/1 -> Mux2/2
  Data Type Conversion23/1 -> Mux2/3
  Data Type Conversion24/1 -> Mux2/4
  Data Type Conversion28/1 -> Mux2/8
  Data Type Conversion27/1 -> Mux2/7
  Data Type Conversion26/1 -> Mux2/6
  Data Type Conversion29/1 -> Mux2/9
  Data Type Conversion32/1 -> Mux2/12
  Data Type Conversion31/1 -> Mux2/11
  Data Type Conversion30/1 -> Mux2/10
  Data Type Conversion33/1 -> Mux2/13
  Data Type Conversion34/1 -> Mux2/14
  Data Type Conversion35/1 -> Mux2/15
  Data Type Conversion37/1 -> Mux2/16

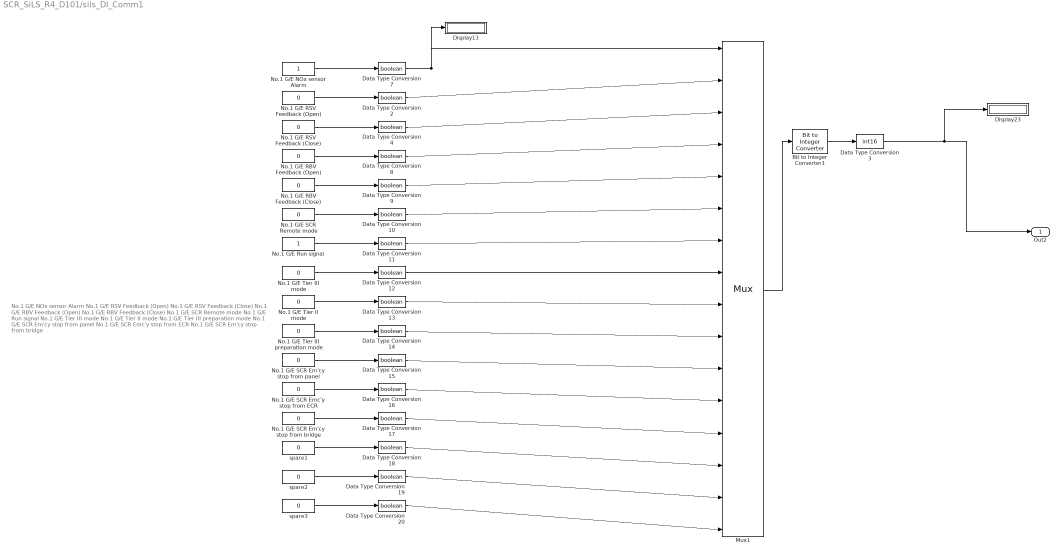
== system SCR_SiLS_R4_D101/sils_DI_Comm1 ==
  note: No.1 G/E NOx sensor Alarm
      |
      | No.1 G/E RSV Feedback (Open)
      |
      | No.1 G/E RSV Feedback (Close)
      |
      | No.1 G/E RBV Feedback (Open)
      |
      | No.1 G/E RBV Feedback (Close)
      |
      | No.1 G/E SCR Remote mode
      |
      | No.1 G/E Run signal
      |
      | No.1 G/E Tier III mode
      |
      | No.1 G/E Tier II mode
      |
      | No.1 G/E Tier III preparation mode
      |
      | No.1 G/E SCR Em'cy stop from panel
      |
      | No.1 G/E SCR Emc'y stop from ECR
      |
      | No.1 G/E SCR Em'cy stop from bridge
  Bit to Integer Converter1 : simulink/Logic and Bit Operations/Bit to Integer Converter  nbits=16  bitOrder=LSB first  signedOutputValues=Unsigned  outDtype=Inherit via internal rule  outDtypeSigned=Inherit via internal rule
  Data Type Conversion{2,4,7..20} (16 alike) : DataTypeConversion  OutDataTypeStr=boolean  SaturateOnIntegerOverflow=off  RndMeth=Floor
  Data Type Conversion3 : DataTypeConversion  OutDataTypeStr=int16  SaturateOnIntegerOverflow=off  RndMeth=Floor
  Display13 : Display
  Display23 : Display
  Mux1 : Mux  Inputs=16
  No.1 G/E NOx sensor Alarm : Constant
  No.1 G/E RBV Feedback (Close) : Constant  Value=0
  No.1 G/E RBV Feedback (Open) : Constant  Value=0
  No.1 G/E RSV Feedback (Close) : Constant  Value=0
  No.1 G/E RSV Feedback (Open) : Constant  Value=0
  No.1 G/E Run signal : Constant
  No.1 G/E SCR Em'cy stop from bridge : Constant  Value=0
  No.1 G/E SCR Em'cy stop from panel : Constant  Value=0
  No.1 G/E SCR Emc'y stop from ECR : Constant  Value=0
  No.1 G/E SCR Remote mode : Constant  Value=0
  No.1 G/E Tier II mode : Constant  Value=0
  No.1 G/E Tier III mode : Constant  Value=0
  No.1 G/E Tier III preparation mode : Constant  Value=0
  spare1 : Constant  Value=0
  spare2 : Constant  Value=0
  spare3 : Constant  Value=0
  Out2 : Outport
  wires:
  No.1 G/E NOx sensor Alarm/1 -> Data Type Conversion7/1
  Data Type Conversion7/1 -> Display13/1, Mux1/1
  Data Type Conversion3/1 -> Out2/1, Display23/1
  Bit to Integer Converter1/1 -> Data Type Conversion3/1
  Mux1/1 -> Bit to Integer Converter1/1
  No.1 G/E RSV Feedback (Open)/1 -> Data Type Conversion2/1
  No.1 G/E RSV Feedback (Close)/1 -> Data Type Conversion4/1
  No.1 G/E RBV Feedback (Open)/1 -> Data Type Conversion8/1
  No.1 G/E RBV Feedback (Close)/1 -> Data Type Conversion9/1
  No.1 G/E SCR Remote mode/1 -> Data Type Conversion10/1
  No.1 G/E Run signal/1 -> Data Type Conversion11/1
  No.1 G/E Tier III mode/1 -> Data Type Conversion12/1
  No.1 G/E Tier II mode/1 -> Data Type Conversion13/1
  No.1 G/E Tier III preparation mode/1 -> Data Type Conversion14/1
  No.1 G/E SCR Em'cy stop from panel/1 -> Data Type Conversion15/1
  No.1 G/E SCR Emc'y stop from ECR/1 -> Data Type Conversion16/1
  No.1 G/E SCR Em'cy stop from bridge/1 -> Data Type Conversion17/1
  spare1/1 -> Data Type Conversion18/1
  spare2/1 -> Data Type Conversion19/1
  spare3/1 -> Data Type Conversion20/1
  Data Type Conversion2/1 -> Mux1/2
  Data Type Conversion4/1 -> Mux1/3
  Data Type Conversion8/1 -> Mux1/4
  Data Type Conversion9/1 -> Mux1/5
  Data Type Conversion10/1 -> Mux1/6
  Data Type Conversion11/1 -> Mux1/7
  Data Type Conversion12/1 -> Mux1/8
  Data Type Conversion13/1 -> Mux1/9
  Data Type Conversion14/1 -> Mux1/10
  Data Type Conversion15/1 -> Mux1/11
  Data Type Conversion16/1 -> Mux1/12
  Data Type Conversion17/1 -> Mux1/13
  Data Type Conversion18/1 -> Mux1/14
  Data Type Conversion19/1 -> Mux1/15
  Data Type Conversion20/1 -> Mux1/16

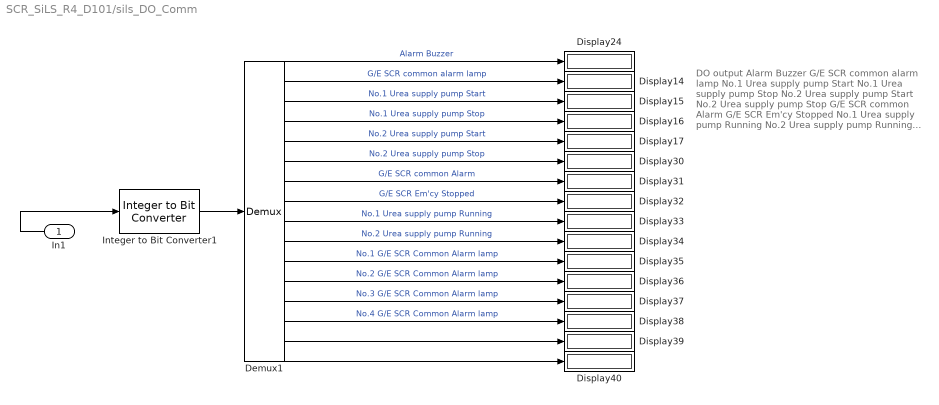
== system SCR_SiLS_R4_D101/sils_DO_Comm ==
  note: DO output
      | Alarm Buzzer
      |
      | G/E SCR common alarm lamp
      |
      | No.1 Urea supply pump Start
      |
      | No.1 Urea supply pump Stop
      |
      | No.2 Urea supply pump Start
      |
      | No.2 Urea supply pump Stop
      |
      | G/E SCR common Alarm
      |
      | G/E SCR Em'cy Stopped
      |
      | No.1 Urea supply pump Running
      |
      | No.2 Urea supply pump Running
      |
      | No.1 G/E SCR Common Alarm lamp
      |
      | No.2 G/E SCR Common Alarm lamp
      |
      | No.3 G/E SCR Common Alarm lamp
      |
      | No.4 G/E SCR Common Alarm lamp
      |
      | ​
      |
      | ​
  In1 : Inport
  Demux1 : Demux  Outputs=16
  Display{14..17,24,30..40} (16 alike) : Display
  Integer to Bit Converter1 : simulink/Logic and Bit Operations/Integer to Bit Converter  nbits=16  signedInputValues=Unsigned  bitOrder=LSB first  outDtype=boolean
  wires:
  Demux1/7 -> Display31/1  "G/E SCR common Alarm"
  Demux1/8 -> Display32/1  "G/E SCR Em'cy Stopped"
  Demux1/9 -> Display33/1  "No.1 Urea supply pump Running"
  Integer to Bit Converter1/1 -> Demux1/1
  In1/1 -> Integer to Bit Converter1/1
  Demux1/1 -> Display24/1  "Alarm Buzzer"
  Demux1/3 -> Display15/1  "No.1 Urea supply pump Start"
  Demux1/5 -> Display17/1  "No.2 Urea supply pump Start"
  Demux1/4 -> Display16/1  "No.1 Urea supply pump Stop"
  Demux1/6 -> Display30/1  "No.2 Urea supply pump Stop"
  Demux1/16 -> Display40/1
  Demux1/2 -> Display14/1  "G/E SCR common alarm lamp"
  Demux1/15 -> Display39/1
  Demux1/10 -> Display34/1  "No.2 Urea supply pump Running"
  Demux1/13 -> Display37/1  "No.3 G/E SCR Common Alarm lamp"
  Demux1/14 -> Display38/1  "No.4 G/E SCR Common Alarm lamp"
  Demux1/12 -> Display36/1  "No.2 G/E SCR Common Alarm lamp"
  Demux1/11 -> Display35/1  "No.1 G/E SCR Common Alarm lamp"

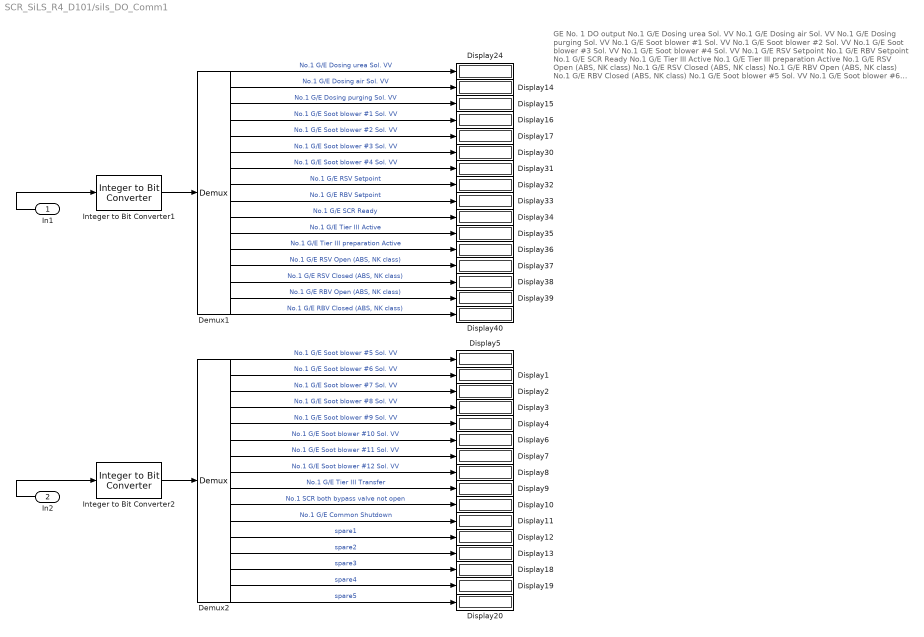
== system SCR_SiLS_R4_D101/sils_DO_Comm1 ==
  note: GE No. 1 DO output
      |
      | No.1 G/E Dosing urea Sol. VV
      |
      | No.1 G/E Dosing air Sol. VV
      |
      | No.1 G/E Dosing purging Sol. VV
      |
      | No.1 G/E Soot blower #1 Sol. VV
      |
      | No.1 G/E Soot blower #2 Sol. VV
      |
      | No.1 G/E Soot blower #3 Sol. VV
      |
      | No.1 G/E Soot blower #4 Sol. VV
      |
      | No.1 G/E RSV Setpoint
      |
      | No.1 G/E RBV Setpoint
      |
      | No.1 G/E SCR Ready
      |
      | No.1 G/E Tier III Active
      |
      | No.1 G/E Tier III preparation Active
      |
      | No.1 G/E RSV Open (ABS, NK class)
      |
      | No.1 G/E RSV Closed (ABS, NK class)
      |
      | No.1 G/E RBV Open (ABS, NK class)
      |
      | No.1 G/E RBV Closed (ABS, NK class)
      |
      | No.1 G/E Soot blower #5 Sol. VV
      |
      | No.1 G/E Soot blower #6 Sol. VV
      |
      | No.1 G/E Soot blower #7 Sol. VV
      |
      | No.1 G/E Soot blower #8 Sol. VV
      |
      | No.1 G/E Soot blower #9 Sol. VV
      |
      | No.1 G/E Soot blower #10 Sol. VV
      |
      | No.1 G/E Soot blower #11 Sol. VV
      |
      | No.1 G/E Soot blower #12 Sol. VV
      |
      | No.1 G/E Tier III Transfer
      |
      | No.1 SCR both bypass valve not open
      |
      | No.# G/E Common Shutdown
  In1 : Inport
  In2 : Inport  Port=2
  Demux1 : Demux  Outputs=16
  Demux2 : Demux  Outputs=16
  Display{1..20,24,30..40} (32 alike) : Display
  Integer to Bit Converter1 : simulink/Logic and Bit Operations/Integer to Bit Converter  nbits=16  signedInputValues=Unsigned  bitOrder=LSB first  outDtype=boolean
  Integer to Bit Converter2 : simulink/Logic and Bit Operations/Integer to Bit Converter  nbits=16  signedInputValues=Unsigned  bitOrder=LSB first  outDtype=boolean
  wires:
  Demux1/7 -> Display31/1  "No.1 G/E Soot blower #4 Sol. VV"
  Demux1/8 -> Display32/1  "No.1 G/E RSV Setpoint"
  Demux1/9 -> Display33/1  "No.1 G/E RBV Setpoint"
  Integer to Bit Converter1/1 -> Demux1/1
  In1/1 -> Integer to Bit Converter1/1
  Demux1/1 -> Display24/1  "No.1 G/E Dosing urea Sol. VV"
  Demux1/3 -> Display15/1  "No.1 G/E Dosing purging Sol. VV"
  Demux1/5 -> Display17/1  "No.1 G/E Soot blower #2 Sol. VV"
  Demux1/4 -> Display16/1  "No.1 G/E Soot blower #1 Sol. VV"
  Demux1/6 -> Display30/1  "No.1 G/E Soot blower #3 Sol. VV"
  Demux1/16 -> Display40/1  "No.1 G/E RBV Closed (ABS, NK class)"
  Demux1/2 -> Display14/1  "No.1 G/E Dosing air Sol. VV"
  Demux1/15 -> Display39/1  "No.1 G/E RBV Open (ABS, NK class)"
  Demux1/10 -> Display34/1  "No.1 G/E SCR Ready"
  Demux1/13 -> Display37/1  "No.1 G/E RSV Open (ABS, NK class)"
  Demux1/14 -> Display38/1  "No.1 G/E RSV Closed (ABS, NK class)"
  Demux1/12 -> Display36/1  "No.1 G/E Tier III preparation Active"
  Demux1/11 -> Display35/1  "No.1 G/E Tier III Active"
  Demux2/1 -> Display5/1  "No.1 G/E Soot blower #5 Sol. VV"
  Demux2/13 -> Display13/1  "spare2"
  In2/1 -> Integer to Bit Converter2/1
  Demux2/10 -> Display10/1  "No.1 SCR both bypass valve not open"
  Demux2/11 -> Display11/1  "No.1 G/E Common Shutdown"
  Demux2/2 -> Display1/1  "No.1 G/E Soot blower #6 Sol. VV"
  Demux2/5 -> Display4/1  "No.1 G/E Soot blower #9 Sol. VV"
  Demux2/14 -> Display18/1  "spare3"
  Demux2/15 -> Display19/1  "spare4"
  Integer to Bit Converter2/1 -> Demux2/1
  Demux2/8 -> Display8/1  "No.1 G/E Soot blower #12 Sol. VV"
  Demux2/4 -> Display3/1  "No.1 G/E Soot blower #8 Sol. VV"
  Demux2/6 -> Display6/1  "No.1 G/E Soot blower #10 Sol. VV"
  Demux2/12 -> Display12/1  "spare1"
  Demux2/9 -> Display9/1  "No.1 G/E Tier III Transfer"
  Demux2/16 -> Display20/1  "spare5"
  Demux2/3 -> Display2/1  "No.1 G/E Soot blower #7 Sol. VV"
  Demux2/7 -> Display7/1  "No.1 G/E Soot blower #11 Sol. VV"
